simulink model "AD_Vehicle_part4"  (R2021a)
settings: Solver=VariableStepAuto  StartTime=0.0  StopTime=100  RelTol=1e-3
libraries: vrlib x2, simulink x1, mpcadaslib x1
settings Model: Creator=admin  LastModifiedBy=admin

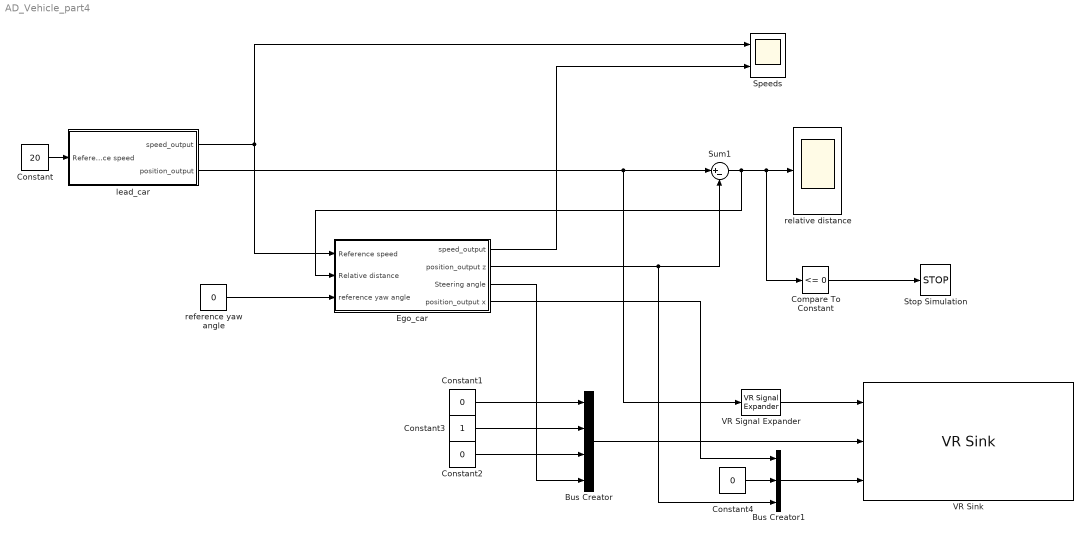
== system AD_Vehicle_part4 ==
  Bus Creator : BusCreator  Inputs=4
  Bus Creator1 : BusCreator  Inputs=3
  Compare To Constant : simulink/Logic and Bit Operations/Compare To Constant  relop=<=  const=0  OutDataTypeStr=boolean
  Constant : Constant  Value=20
  Constant1 : Constant  Value=0
  Constant2 : Constant  Value=0
  Constant3 : Constant
  Constant4 : Constant  Value=0
  Ego_car : Subsystem  mask{Pos_Z=0, Speed=30, Pos_X=0}
      mask prompts: Pos_Z "Initial Position Z"; Speed "Initial Speed"; Pos_X "Initial position x"
      mask TypeOptions Pos_Z: initial_position z/Value
      mask TypeOptions Speed: initial_speed/Value
      mask TypeOptions Pos_X: initial_position x/Value
  Speeds : Scope  NumInputPorts=2
  Stop Simulation : Stop
  Sum1 : Sum  Inputs=|+-
  VR Signal Expander : vrlib/VR Signal Expander  outwidth=3  outidx=[3]
  VR Sink : vrlib/VR Sink  InstantiateOnLoad=on  SampleTime=0.05  ViewEnable=on  RemoteChange=off  RemoteView=off  FieldsWritten=Car_Red.translation.3.1.1.double#Car_Blue.rotation.4.1.1.double#Car_Blue.translation.3.1.1.double  WorldFileName=PlatoonWorld.WRL  AutoView=off  VideoDimensions=[]  AllowVariableSize=off  FigureProperties="{'Position', 'Name', 'Viewpoint', 'CameraBound', 'CameraDirection', 'CameraPosition', 'CameraUpVector', 'ZoomFactor', 'Antialiasing', 'Headlight', 'Lighting', 'NavPanel', 'Sound', 'StatusBar', 'Stereo3D', 'Stereo3DCameraOffset', 'Stereo3DHIT', 'ToolBar', 'Textures', 'Transparency', 'Triad', 'Wireframe', 'NavZones', 'NavMode', 'NavSpeed', 'CaptureFileFormat', 'CaptureFileName', 'Record2DCompressMethod', 'Record2DCompressQuality', 'Record2D', 'Record2DFileName', 'Record2DFPS'; [1.0000000000000000e+00   6.7000000000000000e+01   1.2800000000000000e+03   6.3400000000000000e+02], '', 'Top Cam', 'on', [-3.1410752802896701e-02   0.0000000000000000e+00  -9.9950656056293863e-01], [1.4134838761303510e+00   0.0000000000000000e+00   1.6597779522533207e+02], [0.0000000000000000e+00   1.0000000000000000e+00   0.0000000000000000e+00], [1.0000000000000000e+00], 'on', 'on', 'on', 'halfbar', 'on', 'on', 'off', [1.0000000149011612e-01], [0.0000000000000000e+00], 'on', 'on', 'on', 'none', 'off', 'off', 'walk', 'normal', 'tif', '%f_anim_%n.tif', 'auto', [7.5000000000000000e+01], 'off', '%f_anim_%n.avi', 'auto'}"
  lead_car : Subsystem  mask{Pos=100, Speed=20}
      mask prompts: Pos "Initial Position"; Speed "Initial Speed"
      mask TypeOptions Pos: initial_position/Value
      mask TypeOptions Speed: initial_speed/Value
  reference yaw angle : Constant  Value=0
  relative distance : Scope
  wires:
  Constant/1 -> lead_car/1(Reference speed)
  Ego_car/1(speed_output) -> Speeds/2
  lead_car/1(speed_output) -> Speeds/1, Ego_car/1(Reference speed)
  lead_car/2(position_output) -> VR Signal Expander/1, Sum1/1
  Sum1/1 -> Ego_car/2(Relative distance), Compare To Constant/1, relative distance/1
  Ego_car/2(position_output z) -> Bus Creator1/3, Sum1/2
  Compare To Constant/1 -> Stop Simulation/1
  reference yaw angle/1 -> Ego_car/3(reference yaw angle)
  VR Signal Expander/1 -> VR Sink/1
  Bus Creator1/1 -> VR Sink/3
  Ego_car/3(Steering angle) -> Bus Creator/4
  Bus Creator/1 -> VR Sink/2
  Constant1/1 -> Bus Creator/1
  Constant2/1 -> Bus Creator/3
  Constant3/1 -> Bus Creator/2
  Constant4/1 -> Bus Creator1/2
  Ego_car/4(position_output x) -> Bus Creator1/1

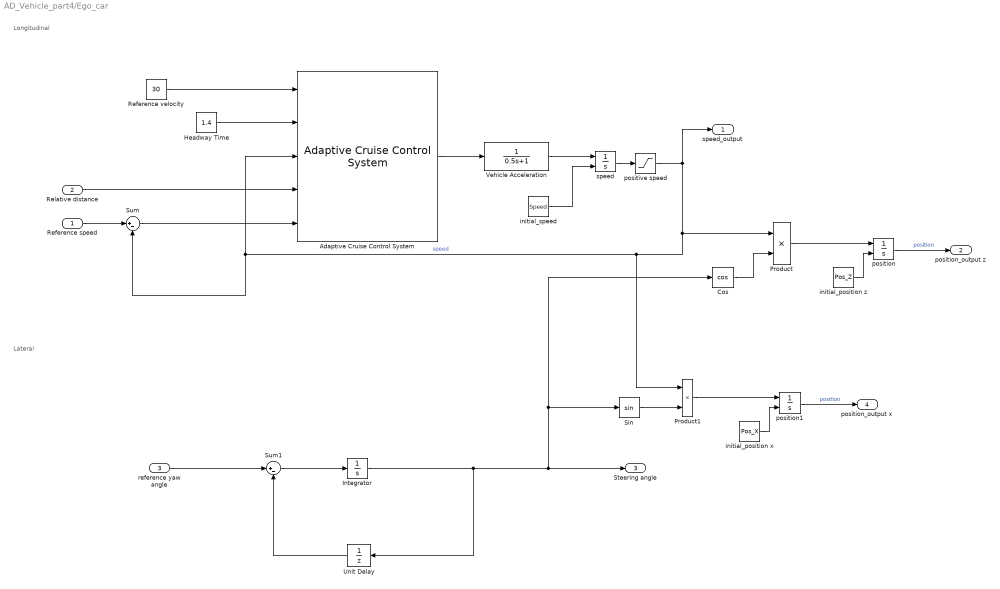
== system AD_Vehicle_part4/Ego_car ==
  note: Lateral
  note: Longitudinal
  Reference speed : Inport
  Relative distance : Inport  Port=2
  reference yaw angle : Inport  Port=3
  Adaptive Cruise Control System : mpcadaslib/Adaptive Cruise Control System  EgoModel=tf(1,[0.5,1,0])  InitialEgoVelocity=30  DefaultSpacing=5  MaxVelocity=50  MinAcceleration=-3  amin_ext=off  MaxAcceleration=2  amax_ext=off  Ts=0.5  PredictionHorizon=200  ControllerBehavior=0.59  suboptimal=off  maxiter=10  datatypeopt=double  optmode=off  trackmode=off
  Cos : Trigonometry  Operator=cos
  Headway Time : Constant  Value=1.4
  Integrator : Integrator
  Product : Product
  Product1 : Product
  Reference velocity : Constant  Value=30
  Sin : Trigonometry
  Sum : Sum  Inputs=|+-
  Sum1 : Sum  Inputs=|+-
  Unit Delay : UnitDelay  SampleTime=-1  HasFrameUpgradeWarning=on
  Vehicle Acceleration : TransferFcn  Denominator=[0.5 1]
  initial_position x : Constant  Value=Pos_X
  initial_position z : Constant  Value=Pos_Z
  initial_speed : Constant  Value=Speed
  position : Integrator  InitialConditionSource=external
  position1 : Integrator  InitialConditionSource=external
  positive speed : Saturate  UpperLimit=220  LowerLimit=0
  speed : Integrator  InitialConditionSource=external
  speed_output : Outport
  position_output z : Outport  Port=2
  Steering angle : Outport  Port=3
  position_output x : Outport  Port=4
  wires:
  Adaptive Cruise Control System/1 -> Vehicle Acceleration/1
  positive speed/1 -> Product/1, Product1/1, Sum/2, Adaptive Cruise Control System/3, speed_output/1  "speed"
  position/1 -> position_output z/1  "position"
  speed/1 -> positive speed/1
  initial_position z/1 -> position/2
  initial_speed/1 -> speed/2
  Reference speed/1 -> Sum/1
  Vehicle Acceleration/1 -> speed/1
  Sum/1 -> Adaptive Cruise Control System/5
  Relative distance/1 -> Adaptive Cruise Control System/4
  Headway Time/1 -> Adaptive Cruise Control System/2
  Reference velocity/1 -> Adaptive Cruise Control System/1
  Integrator/1 -> Unit Delay/1, Cos/1, Sin/1, Steering angle/1
  reference yaw angle/1 -> Sum1/1
  Sum1/1 -> Integrator/1
  Unit Delay/1 -> Sum1/2
  initial_position x/1 -> position1/2
  position1/1 -> position_output x/1  "position"
  Product/1 -> position/1
  Cos/1 -> Product/2
  Product1/1 -> position1/1
  Sin/1 -> Product1/2

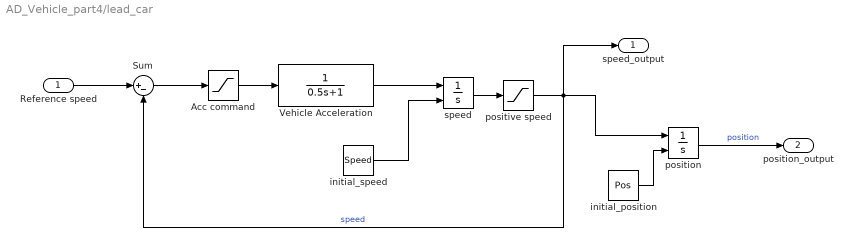
== system AD_Vehicle_part4/lead_car ==
  Reference speed : Inport
  Acc command : Saturate  UpperLimit=2  LowerLimit=-3
  Sum : Sum  Inputs=|+-
  Vehicle Acceleration : TransferFcn  Denominator=[0.5 1]
  initial_position : Constant  Value=Pos
  initial_speed : Constant  Value=Speed
  position : Integrator  InitialConditionSource=external
  positive speed : Saturate  UpperLimit=220  LowerLimit=0
  speed : Integrator  InitialConditionSource=external
  speed_output : Outport
  position_output : Outport  Port=2
  wires:
  Acc command/1 -> Vehicle Acceleration/1
  positive speed/1 -> speed_output/1, Sum/2, position/1  "speed"
  position/1 -> position_output/1  "position"
  speed/1 -> positive speed/1
  initial_position/1 -> position/2
  Sum/1 -> Acc command/1
  initial_speed/1 -> speed/2
  Reference speed/1 -> Sum/1
  Vehicle Acceleration/1 -> speed/1
